simulink model "simulink_model_deney1_2"  (R2014a)
settings: Solver=FixedStepDiscrete  StartTime=0.0  StopTime=1  FixedStep=0.001  RelTol=1e-3
undefined symbols (not defined in the file): High
libraries: simulink_extras x1, dspsrcs4 x1
settings Model: Creator=cya  LastModifiedBy=cya

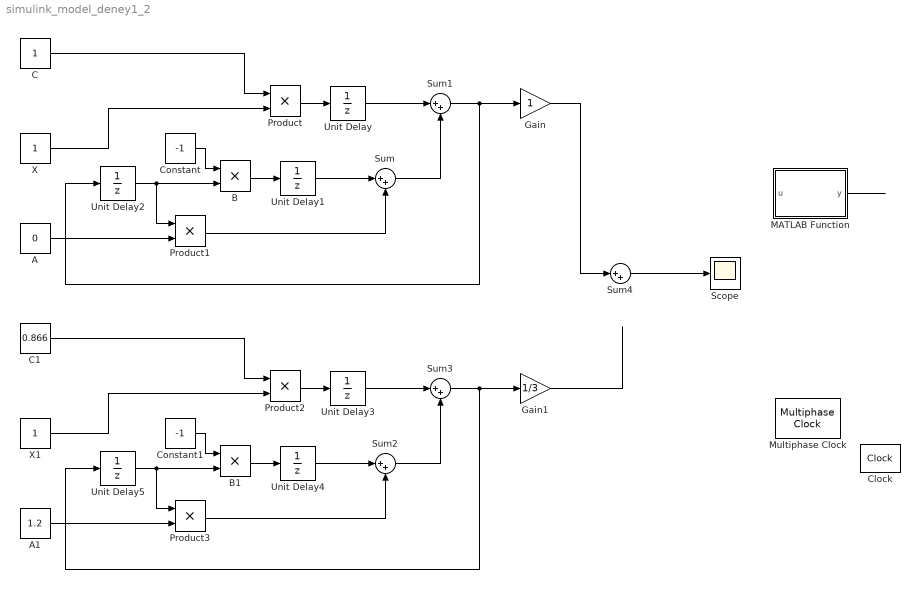
== system simulink_model_deney1_2 ==
  A : Constant  Value=0
  A1 : Constant  Value=1.2
  B : Product
  B1 : Product
  C : Constant
  C1 : Constant  Value=0.866
  Clock : simulink_extras/Flip Flops/Clock  period=2
  Constant : Constant  Value=-1
  Constant1 : Constant  Value=-1
  Gain : Gain
  Gain1 : Gain  Gain=1/3
  MATLAB Function : MATLAB Function  TreatAsAtomicUnit=on
  Multiphase Clock : dspsrcs4/Multiphase Clock  ClkFreq=1  NumPhases=4  StartPhase=1  DutyCycle=3  ActiveLevel=High (1)  DataType=Logical
  Product{,1..3} (4 alike) : Product
  Scope : Scope
  Sum{,1..4} (5 alike) : Sum  Inputs=|++
  Unit Delay{,1..5} (6 alike) : UnitDelay  SampleTime=-1
  X : Constant
  X1 : Constant
  wires:
  Sum/1 -> Sum1/2
  Constant/1 -> B/1
  B/1 -> Unit Delay1/1
  Unit Delay1/1 -> Sum/1
  Unit Delay2/1 -> Product1/1, B/2
  Product1/1 -> Sum/2
  A/1 -> Product1/2
  C/1 -> Product/1
  Product/1 -> Unit Delay/1
  X/1 -> Product/2
  Unit Delay/1 -> Sum1/1
  Sum1/1 -> Gain/1, Unit Delay2/1
  Sum2/1 -> Sum3/2
  Constant1/1 -> B1/1
  B1/1 -> Unit Delay4/1
  Unit Delay4/1 -> Sum2/1
  Unit Delay5/1 -> Product3/1, B1/2
  Product3/1 -> Sum2/2
  A1/1 -> Product3/2
  C1/1 -> Product2/1
  Product2/1 -> Unit Delay3/1
  X1/1 -> Product2/2
  Unit Delay3/1 -> Sum3/1
  Sum3/1 -> Gain1/1, Unit Delay5/1
  Gain/1 -> Sum4/1
  Sum4/1 -> Scope/1
  Gain1/1 -> ?
  ? -> MATLAB Function/1(u)
  MATLAB Function/1(y) -> ?

== matlab function simulink_model_deney1_2/MATLAB Function ==
  data: u input; y output
function y = fcn(u)
%#codegen

y = u;
